simulink model "Cuk_Converter"  (R2021a)
settings: Solver=VariableStepAuto  StartTime=0.0  StopTime=0.1  MaxStep=1e-4  RelTol=1e-3
libraries: spsSeriesRLCBranchLib x5, spsCurrentMeasurementLib x4, spsDiodeLib x1, spsIGBTLib x1, spsDCVoltageSourceLib x1, spsVoltageMeasurementLib x1, spspowerguiLib x1
settings Model: Creator=User  LastModifiedBy=User

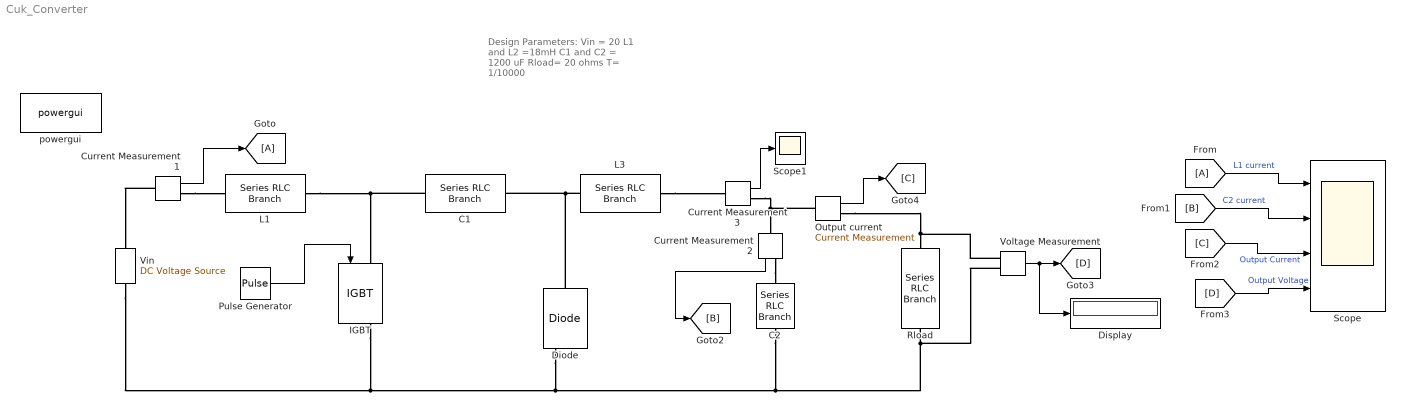
== system Cuk_Converter ==
  note: Design Parameters:
      |
      | Vin = 20
      | L1 and L2 =18mH
      | C1 and C2 = 1200 uF
      | Rload= 20 ohms
      | T= 1/10000
  C1 : spsSeriesRLCBranchLib/Series RLC Branch  LConnTagsString=__new0  RConnTagsString=__new0  BranchType=C  Resistance=1  Inductance=1e-3  SetiL0=off  InitialCurrent=0  Capacitance=1200e-6  Setx0=off  InitialVoltage=0  Measurements=None
  C2 : spsSeriesRLCBranchLib/Series RLC Branch  LConnTagsString=__new0  RConnTagsString=__new0  BranchType=C  Resistance=1  Inductance=1e-3  SetiL0=off  InitialCurrent=0  Capacitance=1200e-6  Setx0=off  InitialVoltage=0  Measurements=None
  Current Measurement1 : spsCurrentMeasurementLib/Current Measurement  PhasorSimulation=off  OutputType=Complex  PSBequivalent=0
  Current Measurement2 : spsCurrentMeasurementLib/Current Measurement  PhasorSimulation=off  OutputType=Complex  PSBequivalent=0
  Current Measurement3 : spsCurrentMeasurementLib/Current Measurement  PhasorSimulation=off  OutputType=Complex  PSBequivalent=0
  Diode : spsDiodeLib/Diode  Ron=0.001  Lon=0  Vf=0.8  IC=0  UseSnubber=0  Rs=500  Cs=250e-9  Measurements=on
  Display : Display
  IGBT : spsIGBTLib/IGBT  Ron=0.001  Lon=0  Vf=1  Tf=1e-6  Tt=2e-6  IC=0  Rs=1e5  Cs=inf  Measurements=on
  L1 : spsSeriesRLCBranchLib/Series RLC Branch  LConnTagsString=__new0  RConnTagsString=__new0  BranchType=L  Resistance=1  Inductance=18e-3  SetiL0=off  InitialCurrent=0  Capacitance=1e-6  Setx0=off  InitialVoltage=0  Measurements=None
  L3 : spsSeriesRLCBranchLib/Series RLC Branch  LConnTagsString=__new0  RConnTagsString=__new0  BranchType=L  Resistance=1  Inductance=18e-3  SetiL0=off  InitialCurrent=0  Capacitance=1e-6  Setx0=off  InitialVoltage=0  Measurements=None
  Output current : spsCurrentMeasurementLib/Current Measurement  PhasorSimulation=off  OutputType=Complex  PSBequivalent=0
  Pulse Generator : DiscretePulseGenerator  PulseType=Time based  Period=1/10000  PulseWidth=80
  Rload : spsSeriesRLCBranchLib/Series RLC Branch  LConnTagsString=__new0  RConnTagsString=__new0  BranchType=R  Resistance=20  Inductance=1e-3  SetiL0=off  InitialCurrent=0  Capacitance=1e-6  Setx0=off  InitialVoltage=0  Measurements=None
  Scope : Scope  NumInputPorts=4
  Scope1 : Scope
  Vin : spsDCVoltageSourceLib/DC Voltage Source  Amplitude=20  Measurements=None
  Voltage Measurement : spsVoltageMeasurementLib/Voltage Measurement  PhasorSimulation=off  OutputType=Complex  PSBequivalent=0
  powergui : spspowerguiLib/powergui  Priority=1  SimulationMode=Continuous  SampleTime=50e-6  frequency=60  Iterations=50  frequencyindice=0  Pbase=100e6  ErrMax=1e-4  UnitsV=kV  UnitsW=MW  buscounter=0  FunctionMessages=off  echomessages=off  EnableUseOfTLC=off  CurrentSourceSwitches=off  DisableSnubberDevices=off  DisableRonSwitches=off  DisableVfSwitches=off  DisplayEquations=off  AutomaticDiscreteSolvers=off  SolverType=Tustin/Backward Euler (TBE)  Interpol=off  ExternalGateDelay=off  methode=off  Ts=100  x0status=blocks  SPID=on  SwTol=0  HookPort=off  NonlinearTolerance=1e-4  nMaxIteration=100  ContinueOnMaxIteration=off  RestoreLinks=warning  ResistiveCurrentMeasurement=off  Frange=[0:2:500]  Ylog=off  Xlog=on  ShowGrid=off  save=off  variable=ZData  structure=0  ZoomFFT=off  StartTime=0.0  cycles=1  DisplayStyle=1  fundamental=60  FreqAxis=off  MaxFrequency=1000  frequencyindicesteady=1  RmsSteady=1  display=off
  wires:
  [B] -> Scope/2  "C2 current"
  Voltage Measurement/1 -> Display/1, [D]
  Output current/1 -> [C]
  Current Measurement1/1 -> [A]
  [C] -> Scope/3  "Output Current"
  [A] -> Scope/1  "L1 current"
  Current Measurement3/1 -> Scope1/1
  Current Measurement2/1 -> [B]
  [D] -> Scope/4  "Output Voltage"
  Pulse Generator/1 -> IGBT/1
  connections:
  Current Measurement3/RConn1 -- Current Measurement2/LConn1 -- Output current/LConn1
  Output current/RConn1 -- Voltage Measurement/LConn1 -- Rload/LConn1
  Rload/RConn1 -- Diode/RConn1 -- IGBT/RConn1 -- Vin/LConn1 -- C2/RConn1 -- Voltage Measurement/LConn2
  L1/RConn1 -- C1/LConn1 -- IGBT/LConn1
  L3/LConn1 -- Current Measurement3/LConn1
  Current Measurement1/LConn1 -- Vin/RConn1
  Current Measurement1/RConn1 -- L1/LConn1
  Current Measurement2/RConn1 -- C2/LConn1
  L3/RConn1 -- Diode/LConn1 -- C1/RConn1
